simulink model "standardize_not"  (Simulink 7.8)
settings: Solver=ode45  StartTime=0.0  StopTime=10.0  RelTol=1e-3
libraries: dspstat3 x2
settings Model: Creator=Leo  LastModifiedBy=Leo

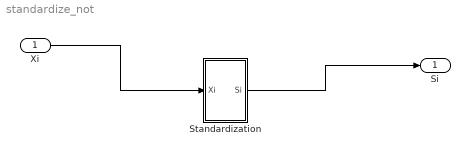
== system standardize_not ==
  Xi : Inport
  Standardization : Subsystem
  Si : Outport
  wires:
  Xi/1 -> Standardization/1(Xi)
  Standardization/1(Si) -> Si/1

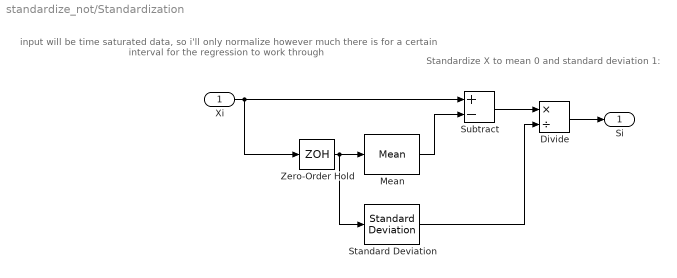
== system standardize_not/Standardization ==
  note: input will be time saturated data,
      | so i'll only normalize however much
      | there is for a certain interval for the
      | regression to work through
  note: Standardize X to mean 0 and standard deviation 1:
  Xi : Inport
  Divide : Product  Inputs=*/
  Mean : dspstat3/Mean  run=off  reset_popup=None  InputProcessing=Columns as channels (frame based)  directionMode=Each column  dimension=1  treatSBRowAsCol=on  roiEnable=off  roiType=Rectangles  roiPortion=Entire ROI  roiOutput=Individual statistics for each ROI  roiFlag=off  outputDataTypeStr=Inherit: Same as accumulator  outputLastDataTypeStr=Inherit: Same as accumulator  outputMin=[]  outputMax=[]  roundingMode=Floor  overflowMode=off
  Standard Deviation : dspstat3/Standard Deviation  run=off  reset_popup=None  InputProcessing=Columns as channels (frame based)  directionMode=Each column  dimension=1  treatSBRowAsCol=on  roiEnable=off  roiType=Rectangles  roiPortion=Entire ROI  roiOutput=Individual statistics for each ROI  roiFlag=off
  Subtract : Sum  Inputs=+-
  Zero-Order Hold : ZeroOrderHold  SampleTime=-1
  Si : Outport
  wires:
  Xi/1 -> Zero-Order Hold/1, Subtract/1
  Zero-Order Hold/1 -> Mean/1, Standard Deviation/1
  Mean/1 -> Subtract/2
  Subtract/1 -> Divide/1
  Standard Deviation/1 -> Divide/2
  Divide/1 -> Si/1
